simulink model "ifelsesf"  (Simulink 7.1)
settings: Solver=FixedStepDiscrete  StartTime=0.0  StopTime=10.0  FixedStep=.01  RelTol=1e-3
settings Model: Creator=ajayaram  LastModifiedBy=ajayaram
settings SolverCC: AutoInsertRateTranBlk=on
settings DataIOCC: SaveOutput=off  SaveTime=off
settings OptimizationCC: InlineParams=on  InlineInvariantSignals=on  EnforceIntegerDowncast=off  StateBitsets=on  DataBitsets=on  UseTempVars=on  OptimizeModelRefInitCode=on  LifeSpan=1
settings DebuggingCC: SaveWithParameterizedLinksMsg=none  SignalResolutionControl=TryResolveAll
settings RTWCC: SystemTargetFile=ert.tlc  GenCodeOnly=on  GenerateMakefile=off  TemplateMakefile=ert_default_tmf  Description=Real-Time Workshop Embedded Coder (no auto configuration)  GenerateReport=on  RTWVerbose=off  ProcessScript=ert_make_rtw_hook  IncludeHyperlinkInReport=on  LaunchReport=on
settings CodeAppCC: GenerateComments=off  IgnoreCustomStorageClasses=off  CustomSymbolStrGlobalVar=rt$N$M  CustomSymbolStrType=$N$M  CustomSymbolStrFcn=$N$M$F  CustomSymbolStrMacro=$N$M  SimulinkBlockComments=off
settings ERTTargetCC: SuppressErrorStatus=on  SupportAbsoluteTime=off  SupportNonFinite=off  SupportComplex=off  InlinedParameterPlacement=NonHierarchical  RootIOFormat=Structure reference  ERTCustomFileTemplate=example_file_process.tlc

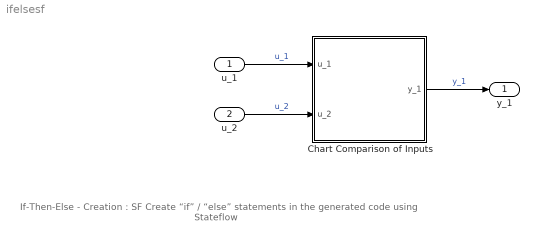
== system ifelsesf ==
  note: If-Then-Else - Creation : SF
      | Create “if” / “else” statements in the
      | generated code using Stateflow
  u_1 : Inport  OutDataType=sfix(16)  OutScaling=2^0
  u_2 : Inport  Port=2  OutDataType=sfix(16)  OutScaling=2^0
  Chart Comparison of Inputs : Stateflow chart
  y_1 : Outport  OutDataType=sfix(16)  OutScaling=2^0
  wires:
  u_1/1 -> Chart Comparison of Inputs/1(u_1)  "u_1"
  u_2/1 -> Chart Comparison of Inputs/2(u_2)  "u_2"
  Chart Comparison of Inputs/1(y_1) -> y_1/1  "y_1"

== stateflow chart Chart Comparison of Inputs ==
  (junction 7) -> (junction 3)
  (junction 4) -> (junction 7) [order 2] : {
      | y_1 = u_2;
      | }
  (junction 4) -> (junction 5) [order 1] : [u_1 > u_2]
  (junction 5) -> (junction 6) : {
      | y_1 = u_1;
      | }
  (junction 6) -> (junction 7)
  (default) -> (junction 4)
  data: u_1 input double; u_2 input double; y_1 output double
